simulink model "Pendulum_extra"  (R2023a)
settings: Solver=ode45  StartTime=0.0  StopTime=tfinal  RelTol=1e-6  EnableMultiTasking=on
values from neighbouring files (symbols this model uses):
  a = g / L    (= 32.6666666667)    [P4.m]    (also in P4_2.m; P4_3_convergence_region.m; P4_4.m; P4_tuning.m)
  b = k / m    (= 0.0333333333333)    [P4.m]    (also in P4_2.m; P4_3_convergence_region.m; P4_4.m; P4_tuning.m)
  c = 1 / (m * L ^ 2)    (= 37.037037037)    [P4.m]    (also in P4_2.m; P4_3_convergence_region.m; P4_4.m; P4_tuning.m)
  dist_amplitude = 0    [P4.m]    (also in P4_2.m; P4_3_convergence_region.m; P4_4.m = 8.5; P4_tuning.m = 2.5)
  flagdist = 0    [P4.m]    (also in P4_2.m; P4_3_convergence_region.m; P4_4.m = 1; P4_tuning.m)
  h = 0.1    [P4.m]    (also in P4_2.m = 0.13; P4_3_convergence_region.m = 0.13; P4_4.m = 0.13; P4_tuning.m = 0.13)
  md = MPCInit(Ad, Bd, Cyd, Czd, Dzd, Ccd, Dcd, Hp, Hw, zblk, Hu, ublk,  	    du_max, du_min ,u_max ,u_min ,z_max,  	    z_min, Q, R, W, V, h, cmode, 'qp_as')    [P4.m]    (also in P4_2.m; P4_3_convergence_region.m; P4_4.m; P4_tuning.m = MPCInit(Ad, Bd, Cyd, Czd, Dzd, Ccd, Dcd, Hp, Hw, zblk, Hu, u)
  square_amplitude = pi / 180    (= 0.0174532925199)    [Pextra.m]
  t_impulse = 0.5    [P4.m]    (also in P4_2.m; P4_3_convergence_region.m; P4_4.m; P4_tuning.m)
  theta_0 = pi / 8    (= 0.392699081699)    [P4.m]    (also in P4_2.m; P4_4.m; P4_tuning.m; Pextra.m = 0.0174532925199)
settings Model: Creator=jakesson  LastModifiedBy=ruipe
settings SolverCC: AlgebraicLoopSolver=TrustRegion
settings DataIOCC: LimitDataPoints=on  SaveFormat=Array  SignalLoggingSaveFormat=ModelDataLogs  ReturnWorkspaceOutputs=off  SignalLoggingName=sigsOut
settings OptimizationCC: BooleanDataType=off  InitFltsAndDblsToZero=on  LifeSpan=inf
settings DebuggingCC: SaveWithParameterizedLinksMsg=none  UnderspecifiedInitializationDetection=Classic  MergeDetectMultiDrivingBlocksExec=none  SignalResolutionControl=TryResolveAllWithWarning  MultiTaskDSMMsg=warning  MultiTaskCondExecSysMsg=none  FcnCallInpInsideContextMsg=warning  UnconnectedInputMsg=warning  UnconnectedOutputMsg=warning  UnconnectedLineMsg=warning  SFUnexpectedBacktrackingDiag=warning  SFNoUnconditionalDefaultTransitionDiag=warning  SFExecutionAtInitializationDiag=none  ArithmeticOperatorsInVariantConditions=warning
settings HardwareCC: ProdBitPerPointer=32  ProdBitPerSizeT=32  ProdBitPerPtrDiffT=32  ProdLargestAtomicFloat=None  ProdIntDivRoundTo=Undefined  ProdEndianess=Unspecified  ProdWordSize=32  ProdHWDeviceType=32-bit Generic  TargetUnknown=on
settings ModelReferenceCC: PropagateSignalLabelsOutOfModel=off
settings SFSimCC: SimUseLocalCustomCode=off  CustomCodeUndefinedFunction=UseInterfaceOnly
settings RTWCC: RTWUseLocalCustomCode=off
settings CodeAppCC: StateflowObjectComments=on
settings GRTTargetCC: TargetFcnLib=ansi_tfl_tmw.mat  TargetLangStandard=C89/C90 (ANSI)  CombineOutputUpdateFcns=off  GRTInterface=on
settings ConfigComp: CovMetricSettings=dw  CovSaveCumulativeToWorkspaceVar=on  CovSaveSingleToWorkspaceVar=on  CovExternalEMLEnable=off

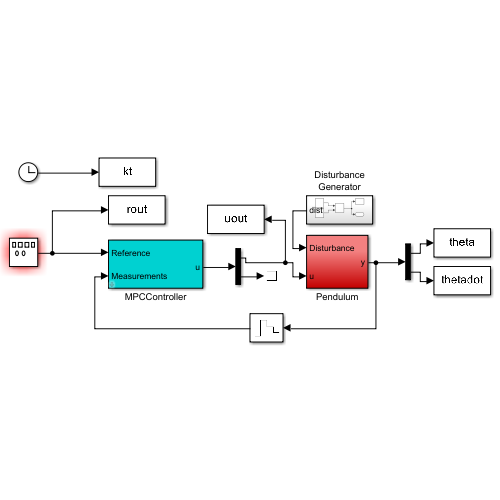
[thumbnail: Simulink's stored preview of the top-level diagram]
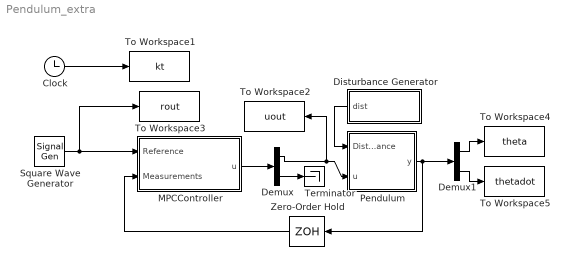
== system Pendulum_extra ==
  Clock : Clock
  Demux : Demux  Outputs=[md.m md.ne]
      settings: DisplayOption=none
  Demux1 : Demux  Outputs=2
  Disturbance Generator : Subsystem
  MPCController : Subsystem  mask{md=md}
      mask prompts: md "MPCData"
  Pendulum : Subsystem
  Square Wave Generator : SignalGenerator  WaveForm=square  Amplitude=square_amplitude  Frequency=2 * pi / 10  Units=rad/sec
  Terminator : Terminator
  To Workspace1 : ToWorkspace  VariableName=kt  SampleTime=-1
  To Workspace2 : ToWorkspace  VariableName=uout  SaveFormat=Structure With Time  SampleTime=-1
  To Workspace3 : ToWorkspace  VariableName=rout  SampleTime=-1
  To Workspace4 : ToWorkspace  VariableName=theta  SaveFormat=Structure With Time  SampleTime=-1
  To Workspace5 : ToWorkspace  VariableName=thetadot  SaveFormat=Structure With Time  SampleTime=-1
  Zero-Order Hold : ZeroOrderHold  SampleTime=h
  wires:
  Demux/2 -> Terminator/1
  MPCController/1(u) -> Demux/1
  Clock/1 -> To Workspace1/1
  Demux/1 -> Pendulum/2(u), To Workspace2/1
  Square Wave Generator/1 -> To Workspace3/1, MPCController/1(Reference)
  Zero-Order Hold/1 -> MPCController/2(Measurements)
  Pendulum/1(y) -> Demux1/1, Zero-Order Hold/1
  Disturbance Generator/1(dist) -> Pendulum/1(Disturbance)
  Demux1/1 -> To Workspace4/1
  Demux1/2 -> To Workspace5/1

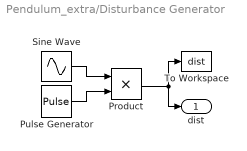
== system Pendulum_extra/Disturbance Generator ==
  Product : Product
  Pulse Generator : DiscretePulseGenerator  PulseType=Time based  Period=10  PulseWidth=t_impulse*10  PhaseDelay=5
  Sine Wave : Sin  Amplitude=dist_amplitude  Frequency=pi/t_impulse  SampleTime=0
  To Workspace : ToWorkspace  VariableName=dist  SaveFormat=Structure With Time  SampleTime=-1
  dist : Outport
  wires:
  Pulse Generator/1 -> Product/2
  Sine Wave/1 -> Product/1
  Product/1 -> To Workspace/1, dist/1

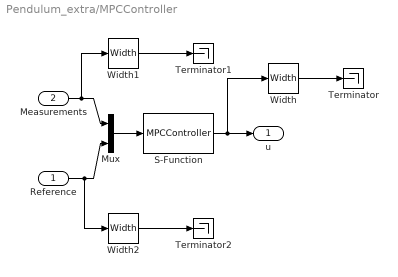
== system Pendulum_extra/MPCController ==
  Reference : Inport
  Measurements : Inport  Port=2
  Mux : Mux  Inputs=2
  S-Function : S-Function  FunctionName=MPCController  Parameters=md  SFunctionDeploymentMode=off  EnableBusSupport=off
  Terminator : Terminator
  Terminator1 : Terminator
  Terminator2 : Terminator
  Width : Width
  Width1 : Width
  Width2 : Width
  u : Outport
  wires:
  Mux/1 -> S-Function/1
  Measurements/1 -> Width1/1, Mux/1
  Reference/1 -> Width2/1, Mux/2
  S-Function/1 -> Width/1, u/1
  Width/1 -> Terminator/1
  Width1/1 -> Terminator1/1
  Width2/1 -> Terminator2/1

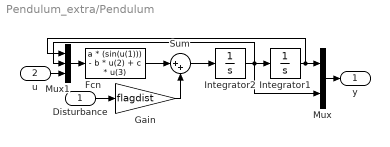
== system Pendulum_extra/Pendulum ==
  Disturbance : Inport
  u : Inport  Port=2
  Fcn : Fcn  Expr=a * (sin(u(1))) - b * u(2) + c * u(3)
  Gain : Gain  Gain=flagdist
  Integrator1 : Integrator  InitialCondition=theta_0
  Integrator2 : Integrator
  Mux : Mux  Inputs=2
  Mux1 : Mux  Inputs=3
  Sum : Sum  Inputs=|++
  y : Outport
  wires:
  Integrator2/1 -> Mux1/2, Mux/2, Integrator1/1
  Mux/1 -> y/1
  Mux1/1 -> Fcn/1
  Integrator1/1 -> Mux/1, Mux1/1
  u/1 -> Mux1/3
  Fcn/1 -> Sum/1
  Sum/1 -> Integrator2/1
  Disturbance/1 -> Gain/1
  Gain/1 -> Sum/2
